simulink model "SimulationGuidedRecovery"  (R2023b)
settings: Solver=VariableStepAuto  StartTime=0.0  StopTime=600  RelTol=1e-3
libraries: slpidlib x1
settings Model: Creator=Jerry Gao  LastModifiedBy=Jerry Gao

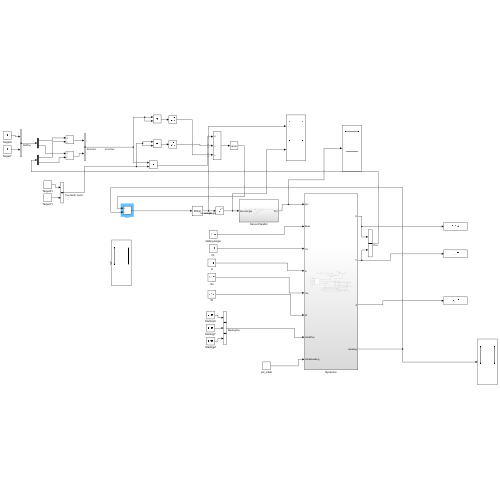
[thumbnail: Simulink's stored preview of the top-level diagram]
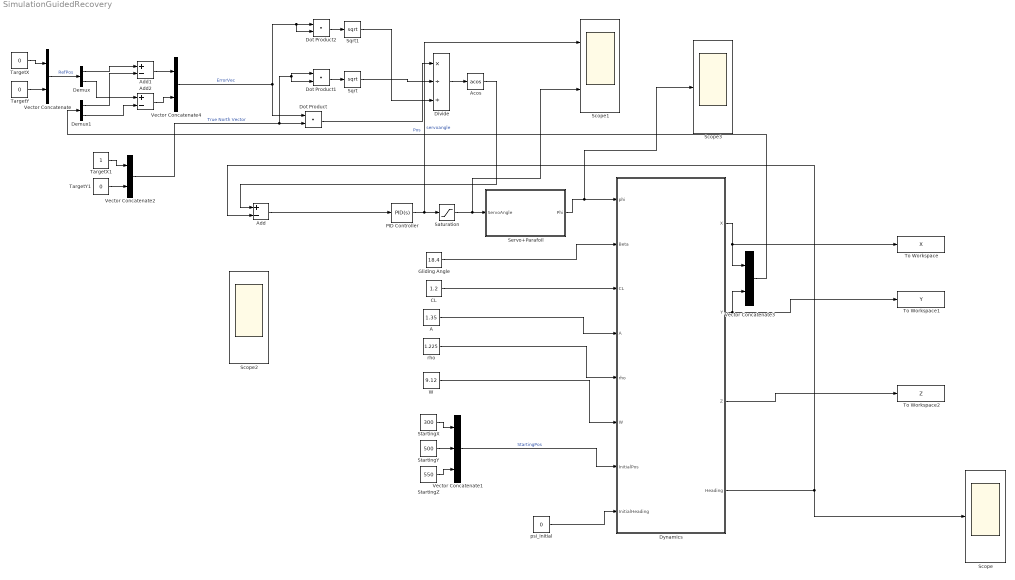
== system SimulationGuidedRecovery ==
  A : Constant  Value=1.35
  Acos : Trigonometry  Operator=acos
  Add : Sum  Inputs=+-
  Add1 : Sum  Inputs=+-
  Add2 : Sum  Inputs=+-
  CL : Constant  Value=1.2
  Demux : Demux  Outputs=2
  Demux1 : Demux  Outputs=2
  Divide : Product  Inputs=*//
  Dot Product : DotProduct  OutDataTypeStr=Inherit: Inherit via internal rule
  Dot Product1 : DotProduct  OutDataTypeStr=Inherit: Inherit via internal rule
  Dot Product2 : DotProduct  OutDataTypeStr=Inherit: Inherit via internal rule
  Dynamics : Subsystem
  Gliding Angle : Constant  Value=18.4
  PID Controller : slpidlib/PID Controller  Controller=PID  Form=Parallel  TimeDomain=Continuous-time  UseExternalTs=off  SampleTime=-1  IntegratorMethod=Forward Euler  FilterMethod=Forward Euler  ControllerParametersSource=internal  P=80.1153937756282  I=0  UseKiTs=off  D=-635.540237142208  N=0.0341829073350393  UseFilter=on  TunerSelectOption=Transfer Function Based (PID Tuner App)  InitialConditionSource=internal  InitialConditionForIntegrator=0  InitialConditionForFilter=0  DifferentiatorICPrevScaledInput=0  ExternalReset=none  TrackingMode=off  Kt=1  LimitOutput=off  SatLimitsSource=internal  UpperSaturationLimit=inf  LowerSaturationLimit=-inf  LinearizeAsGain=on  AntiWindupMode=none  Kb=1  LimitIntegrator=off  UpperIntegratorSaturationLimit=inf  LowerIntegratorSaturationLimit=-inf  POutMin=[]  POutMax=[]  IOutMin=[]  IOutMax=[]  DOutMin=[]  DOutMax=[]  NOutMin=[]  NOutMax=[]  SumOutMin=[]  SumOutMax=[]  SaturationOutMin=[]  SaturationOutMax=[]  PParamMin=[]  PParamMax=[]  IParamMin=[]  IParamMax=[]  DParamMin=[]  DParamMax=[]  NParamMin=[]  NParamMax=[]  KbParamMin=[]  KbParamMax=[]  KtParamMin=[]  KtParamMax=[]  KbOutMin=[]  KbOutMax=[]  KtOutMin=[]  KtOutMax=[]  IntegratorOutMin=[]  IntegratorOutMax=[]  FilterOutMin=[]  FilterOutMax=[]  SumI1OutMin=[]  SumI1OutMax=[]  SumI2OutMin=[]  SumI2OutMax=[]  SumI3OutMin=[]  SumI3OutMax=[]  SumI4OutMin=[]  SumI4OutMax=[]  SumDOutMin=[]  SumDOutMax=[]  DifferentiatorOutMin=[]  DifferentiatorOutMax=[]  FilterDiffOutCoefMin=[]  FilterDiffOutCoefMax=[]  ReciprocalOutMin=[]  ReciprocalOutMax=[]  SumDenOutMin=[]  SumDenOutMax=[]  SumNumOutMin=[]  SumNumOutMax=[]  DivideOutMin=[]  DivideOutMax=[]  UdiffTsProdOutMin=[]  UdiffTsProdOutMax=[]  NTsProdOutMin=[]  NTsProdOutMax=[]  UintegralTsProdOutMin=[]  UintegralTsProdOutMax=[]  UngainTsProdOutMin=[]  UngainTsProdOutMax=[]  ClampingZeroOutDataTypeStr=Inherit: Inherit via back propagation  ClampingZeroOutMin=[]  ClampingZeroOutMax=[]  FilterDenConstantOutDataTypeStr=Inherit: Inherit via back propagation  FilterDenConstantOutMin=[]  FilterDenConstantOutMax=[]  PCopyOutDataTypeStr=Inherit: Inherit via back propagation  PCopyOutMin=[]  PCopyOutMax=[]  NCopyOutDataTypeStr=Inherit: Inherit via back propagation  NCopyOutMin=[]  NCopyOutMax=[]  IntegratorContinuousStateAttributes=''  IntegratorStateMustResolveToSignalObject=off  IntegratorRTWStateStorageClass=Auto  FilterContinuousStateAttributes=''  FilterStateMustResolveToSignalObject=off  FilterRTWStateStorageClass=Auto  ParallelPVariant=InternalParameters  IdealPVariant=Disabled  IVariant=InternalParameters  DVariant=InternalParameters  IntegratorVariant=Continuous  SatVariant=Disabled  AWVariant=Passthrough  PCopyVariant=Disabled  TRVariant=Disabled  FdbkBlocksVariant=Forward  IdealPFdbkVariant=Disabled  SatFdbkVariant=Disabled  DerivativeFilterVariant=ContFilter  NVariant=InternalParameters  NCopyVariant=Disabled  FilterICVariant=InternalICsFilter  IntegratorICVariant=InternalICs  ExternalResetVariant=Disabled  TRSumVariant=Passthrough  SumFdbkVariant=Disabled  SumVariant=Sum_PID  TsampFilterVariant=InternalTs  TsampNgainVariant=Passthrough  TsampIntegralVariant=Disabled_SignalSpec  ExternalSaturationOutDataTypeStr=Inherit: Same as second input
  Saturation : Saturate  UpperLimit=1260  LowerLimit=-1260
  Scope : Scope
  Scope1 : Scope  NumInputPorts=2
  Scope2 : Scope
  Scope3 : Scope
  Servo+Parafoil : Subsystem
  Sqrt : Sqrt
  Sqrt1 : Sqrt
  StartingX : Constant  Value=300
  StartingY : Constant  Value=500
  StartingZ : Constant  Value=550
  TargetX : Constant  Value=0
  TargetX1 : Constant
  TargetY : Constant  Value=0
  TargetY1 : Constant  Value=0
  To Workspace : ToWorkspace  VariableName=X  SaveFormat=Timeseries  SampleTime=-1
  To Workspace1 : ToWorkspace  VariableName=Y  SaveFormat=Timeseries  SampleTime=-1
  To Workspace2 : ToWorkspace  VariableName=Z  SaveFormat=Timeseries  SampleTime=-1
  Vector Concatenate{,2..4} (4 alike) : Concatenate
  Vector Concatenate1 : Concatenate  NumInputs=3
  W : Constant  Value=9.12
  psi_initial : Constant  Value=0
  rho : Constant  Value=1.225
  wires:
  Add/1 -> PID Controller/1
  Gliding Angle/1 -> Dynamics/2(Beta)
  CL/1 -> Dynamics/3(CL)
  A/1 -> Dynamics/4(A)
  rho/1 -> Dynamics/5(rho)
  W/1 -> Dynamics/6(W)
  TargetX/1 -> Vector Concatenate/1
  TargetY/1 -> Vector Concatenate/2
  StartingY/1 -> Vector Concatenate1/2
  StartingZ/1 -> Vector Concatenate1/3
  StartingX/1 -> Vector Concatenate1/1
  Vector Concatenate1/1 -> Dynamics/7(InitialPos)  "StartingPos"
  Servo+Parafoil/1(Phi) -> Scope3/1, Dynamics/1(phi)
  PID Controller/1 -> Saturation/1, Scope1/1  "servoangle"
  psi_initial/1 -> Dynamics/8(InitialHeading)
  TargetY1/1 -> Vector Concatenate2/2
  TargetX1/1 -> Vector Concatenate2/1
  Vector Concatenate2/1 -> Dot Product1/2, Dot Product1/1, Dot Product/2  "True North Vector"
  Dynamics/1(X) -> To Workspace/1, Vector Concatenate3/1
  Dynamics/2(Y) -> To Workspace1/1, Vector Concatenate3/2
  Vector Concatenate3/1 -> Demux1/1  "Pos"
  Dot Product/1 -> Divide/1
  Sqrt/1 -> Divide/2
  Sqrt1/1 -> Divide/3
  Divide/1 -> Acos/1
  Dynamics/4(Heading) -> Scope/1, Add/2
  Acos/1 -> Add/1
  Vector Concatenate/1 -> Demux/1  "RefPos"
  Demux/1 -> Add1/1
  Demux1/1 -> Add1/2
  Demux/2 -> Add2/1
  Demux1/2 -> Add2/2
  Add1/1 -> Vector Concatenate4/1
  Add2/1 -> Vector Concatenate4/2
  Vector Concatenate4/1 -> Dot Product2/2, Dot Product2/1, Dot Product/1  "ErrorVec"
  Dot Product1/1 -> Sqrt/1
  Dot Product2/1 -> Sqrt1/1
  Dynamics/3(Z) -> To Workspace2/1
  Saturation/1 -> Scope1/2, Servo+Parafoil/1(ServoAngle)

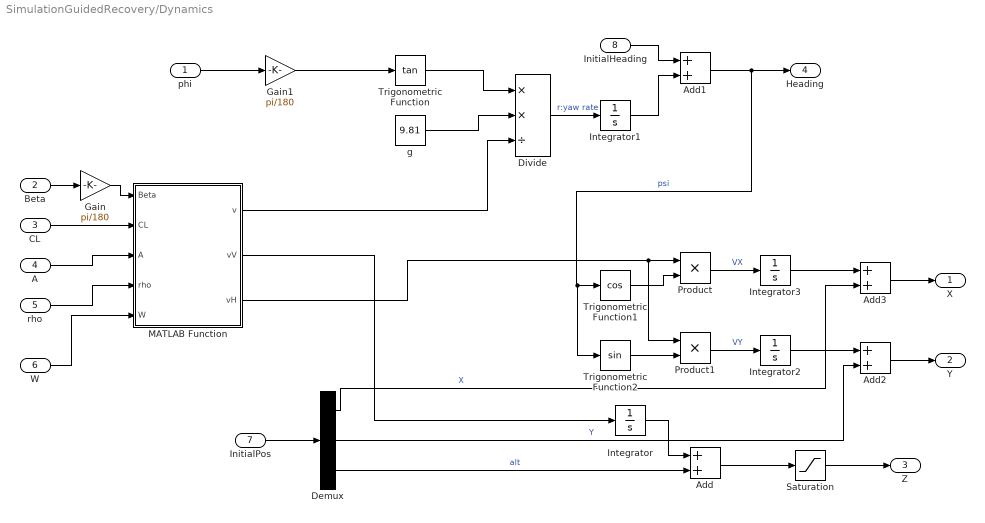
== system SimulationGuidedRecovery/Dynamics ==
  phi : Inport
  Beta : Inport  Port=2
  CL : Inport  Port=3
  A : Inport  Port=4
  rho : Inport  Port=5
  W : Inport  Port=6
  InitialPos : Inport  Port=7
  InitialHeading : Inport  Port=8
  Add{,1..3} (4 alike) : Sum
  Demux : Demux  Outputs=3
  Divide : Product  Inputs=**/
  Gain : Gain  Gain=pi/180
  Gain1 : Gain  Gain=pi/180
  Integrator{,1..3} (4 alike) : Integrator
  MATLAB Function : MATLAB Function  TreatAsAtomicUnit=on
  Product : Product
  Product1 : Product
  Saturation : Saturate  UpperLimit=1000  LowerLimit=0
  Trigonometric Function : Trigonometry  Operator=tan
  Trigonometric Function1 : Trigonometry  Operator=cos
  Trigonometric Function2 : Trigonometry
  g : Constant  Value=9.81
  X : Outport
  Y : Outport  Port=2
  Z : Outport  Port=3
  Heading : Outport  Port=4
  wires:
  Beta/1 -> Gain/1
  CL/1 -> MATLAB Function/2(CL)
  A/1 -> MATLAB Function/3(A)
  rho/1 -> MATLAB Function/4(rho)
  W/1 -> MATLAB Function/5(W)
  Gain/1 -> MATLAB Function/1(Beta)
  MATLAB Function/2(vV) -> Integrator/1
  MATLAB Function/1(v) -> Divide/3
  InitialPos/1 -> Demux/1
  Demux/3 -> Add/2  "alt"
  Demux/2 -> Add2/2  "Y"
  Demux/1 -> Add3/2  "X"
  Integrator/1 -> Add/1
  Add/1 -> Saturation/1
  phi/1 -> Gain1/1
  g/1 -> Divide/2
  Trigonometric Function/1 -> Divide/1
  Divide/1 -> Integrator1/1  "r:yaw rate"
  Integrator1/1 -> Add1/2
  InitialHeading/1 -> Add1/1
  Add1/1 -> Trigonometric Function2/1, Trigonometric Function1/1, Heading/1  "psi"
  Trigonometric Function1/1 -> Product/2
  Product/1 -> Integrator3/1  "VX"
  Trigonometric Function2/1 -> Product1/2
  MATLAB Function/3(vH) -> Product1/1, Product/1
  Product1/1 -> Integrator2/1  "VY"
  Integrator3/1 -> Add3/1
  Integrator2/1 -> Add2/1
  Add2/1 -> Y/1
  Add3/1 -> X/1
  Saturation/1 -> Z/1
  Gain1/1 -> Trigonometric Function/1

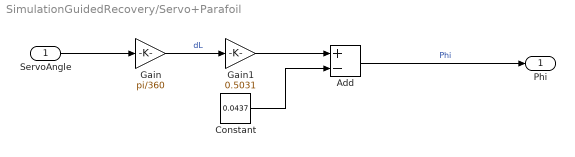
== system SimulationGuidedRecovery/Servo+Parafoil ==
  ServoAngle : Inport
  Add : Sum  Inputs=+-
  Constant : Constant  Value=0.0437
  Gain : Gain  Gain=pi/360
  Gain1 : Gain  Gain=0.5031
  Phi : Outport
  wires:
  ServoAngle/1 -> Gain/1
  Gain/1 -> Gain1/1  "dL"
  Constant/1 -> Add/2
  Gain1/1 -> Add/1
  Add/1 -> Phi/1  "Phi"

== matlab function SimulationGuidedRecovery/Dynamics/MATLAB Function ==
  data: Beta input; v output; CL input; A input; rho input; W input; vV output; vH output
function [v,vV,vH]= findGlidingSpeed(Beta,CL,A,rho,W)

    L = W/(cos(Beta) + tan(Beta)*sin(Beta));
    v = sqrt(2*L/(rho*A*CL));
    vV = -v*sin(Beta);
    vH = v*cos(Beta);
end
